simulink model "Auto_Coffee2"  (R2017a)
settings: Solver=FixedStepAuto  StartTime=0.0  StopTime=25  FixedStep=0.2  RelTol=1e-3
undefined symbols (not defined in the file): sigbuilder_block
libraries: nesl_utility x12, fl_lib x9
settings Model: Creator=Administrator  LastModifiedBy=Administrator
settings OptimizationCC: DefaultParameterBehavior=Inlined  UseDivisionForNetSlopeComputation=on  UseFloatMulNetSlope=on  InlineInvariantSignals=on  PassReuseOutputArgsAs=Individual arguments  ZeroExternalMemoryAtStartup=off  ZeroInternalMemoryAtStartup=off  NoFixptDivByZeroProtection=on  EfficientFloat2IntCast=on  LifeSpan=1
settings DebuggingCC: ParameterTunabilityLossMsg=error
settings HardwareCC: ProdBitPerPointer=32  ProdBitPerSizeT=32  ProdBitPerPtrDiffT=32  ProdLargestAtomicInteger=Long  ProdWordSize=32  ProdHWDeviceType=ARM Compatible->ARM 7
settings SFSimCC: MATLABDynamicMemAlloc=off
settings RTWCC: SystemTargetFile=ert.tlc  TemplateMakefile=ert_default_tmf  Description=Embedded Coder  GenerateReport=on  IncludeHyperlinkInReport=on  LaunchReport=on  GenerateTraceInfo=on  GenerateTraceReport=on  GenerateTraceReportSl=on  GenerateTraceReportSf=on  GenerateTraceReportEml=on  GenerateCodeMetricsReport=on
settings CodeAppCC: ForceParamTrailComments=on  IgnoreCustomStorageClasses=off  OperatorAnnotations=on  SimulinkDataObjDesc=on  SFDataObjDesc=on  MATLABFcnDesc=on  CustomSymbolStrGlobalVar=rt$N$M  CustomSymbolStrType=$N$M  CustomSymbolStrFcn=$N$M$F  CustomSymbolStrMacro=$N$M  InsertBlockDesc=on  MATLABSourceComments=on
settings ERTTargetCC: TargetLangStandard=C99 (ISO)  GenerateSampleERTMain=on  IncludeMdlTerminateFcn=off  CombineSignalStateStructs=on  SupportComplex=off  SupportContinuousTime=on  SupportNonInlinedSFcns=on  InlinedParameterPlacement=NonHierarchical  ERTCustomFileTemplate=example_file_process.tlc  ERTFilePackagingFormat=CompactWithDataFile

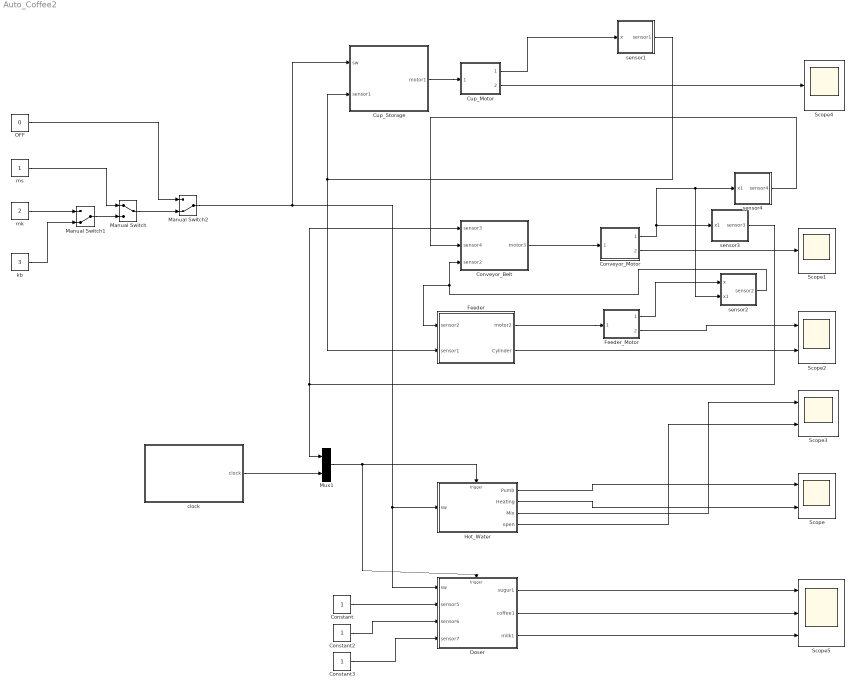
== system Auto_Coffee2 ==
  Constant : Constant
  Constant2 : Constant
  Constant3 : Constant
  Conveyor_Belt : Stateflow chart  TreatAsAtomicUnit=on
  Conveyor_Motor : Subsystem
  Cup_Motor : Subsystem
  Cup_Storage : Stateflow chart  TreatAsAtomicUnit=on
  Doser : Stateflow chart  TreatAsAtomicUnit=on
  Feeder : Stateflow chart  TreatAsAtomicUnit=on
  Feeder_Motor : Subsystem
  Hot_Water : Stateflow chart  TreatAsAtomicUnit=on
  Manual Switch : ManualSwitch
  Manual Switch1 : ManualSwitch  CurrentSetting=0
  Manual Switch2 : ManualSwitch  CurrentSetting=0
  Mux1 : Mux  Inputs=2
  OFF : Constant  Value=0
  Scope : Scope  NumInputPorts=2
  Scope1 : Scope
  Scope2 : Scope  NumInputPorts=2
  Scope3 : Scope  NumInputPorts=2
  Scope4 : Scope
  Scope5 : Scope  NumInputPorts=3
  clock : Subsystem  Tag=STV Subsys  LoadFcn=sigbuilder_block('load');  StartFcn=sigbuilder_block('start');  StopFcn=sigbuilder_block('stop');  ClipboardFcn=sigbuilder_block('clipboard');  mask(Sigbuilder block){tuvar=[0:10]}
      mask help: Simulink:masks:SigbuilderBlock_MD
      mask init:
      | if ~strcmp(get_param(bdroot(gcbh),'SimulationStatus'),'stopped') tuvar = sigbuilder_block('maskInit'); end
      settings: CopyFcn=sigbuilder_block('copy');  DeleteFcn=sigbuilder_block('delete');  ModelCloseFcn=sigbuilder_block('modelClose');  PreSaveFcn=sigbuilder_block('preSave');  PauseFcn=sigbuilder_block('pause');  ContinueFcn=sigbuilder_block('continue');  NameChangeFcn=sigbuilder_block('namechange');  OpenFcn=sigbuilder_block('open',[527.25 182.25 550.5 358.5 ]);  CloseFcn=sigbuilder_block('close');
      mask Display: plot(0, 0, 100, 100,[2, 2, 32, 32, 2], [68, 8, 8, 68, 68],[32, 2], [38, 38], [32, 19, 2],[53, 60, 44], [32, 17, 17, 2],[16, 16, 31, 31]);txt = getActiveGroup(gcbh);text(2, 100, txt,'verticalAlignment', 'top');
  kb : Constant  Value=3
  mk : Constant  Value=2
  ms : Constant
  sensor1 : Stateflow chart  TreatAsAtomicUnit=on
  sensor2 : Stateflow chart  TreatAsAtomicUnit=on
  sensor3 : Stateflow chart  TreatAsAtomicUnit=on
  sensor4 : Stateflow chart  TreatAsAtomicUnit=on
  wires:
  Hot_Water/1(Pumb) -> Scope/1
  Hot_Water/2(Heating) -> Scope/2
  Conveyor_Belt/1(motor3) -> Conveyor_Motor/1(motor3)
  Feeder/1(motor2) -> Feeder_Motor/1(motor2)
  Feeder/2(Cylinder) -> Scope2/2
  Cup_Storage/1(motor1) -> Cup_Motor/1(motor3)
  Constant/1 -> Doser/2(sensor5)
  Constant3/1 -> Doser/4(sensor7)
  Constant2/1 -> Doser/3(sensor6)
  clock/1(clock) -> Mux1/2
  Mux1/1 -> Hot_Water/Trigger, Doser/Trigger
  Manual Switch/1 -> Manual Switch2/2
  Manual Switch1/1 -> Manual Switch/2
  OFF/1 -> Manual Switch2/1
  ms/1 -> Manual Switch/1
  mk/1 -> Manual Switch1/1
  kb/1 -> Manual Switch1/2
  Doser/1(sugur1) -> Scope5/1
  Doser/2(coffee1) -> Scope5/2
  Doser/3(milk1) -> Scope5/3
  Conveyor_Motor/1(position) -> sensor2/2(x1), sensor4/1(x1), sensor3/1(x1)
  sensor4/1(sensor4) -> Conveyor_Belt/2(sensor4)
  Feeder_Motor/1(position) -> sensor2/1(x)
  sensor2/1(sensor2) -> Feeder/1(sensor2), Conveyor_Belt/3(sensor2)
  Cup_Motor/1(position) -> sensor1/1(x)
  sensor1/1(sensor1) -> Feeder/2(sensor1), Cup_Storage/2(sensor1)
  sensor3/1(sensor3) -> Mux1/1, Conveyor_Belt/1(sensor3)
  Manual Switch2/1 -> Hot_Water/1(sw), Doser/1(sw), Cup_Storage/1(sw)
  Hot_Water/3(Mix) -> Scope3/1
  Hot_Water/4(open) -> Scope3/2
  Feeder_Motor/2(scope1) -> Scope2/1
  Conveyor_Motor/2(scope1) -> Scope1/1
  Cup_Motor/2(scope1) -> Scope4/1

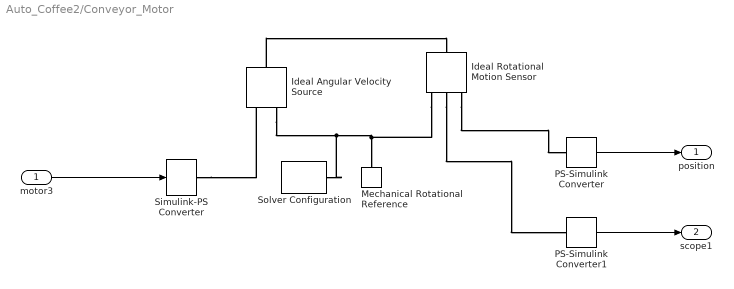
== system Auto_Coffee2/Conveyor_Motor ==
  motor3 : Inport
  Ideal Angular Velocity Source : fl_lib/Mechanical/Mechanical Sources/Ideal Angular Velocity Source
  Ideal Rotational Motion Sensor : fl_lib/Mechanical/Mechanical Sensors/Ideal Rotational Motion Sensor  offset=0 rad
  Mechanical Rotational Reference : fl_lib/Mechanical/Rotational Elements/Mechanical Rotational Reference
  PS-Simulink Converter : nesl_utility/PS-Simulink Converter  PhysicalDomain=network_engine_domain  SubClassName=ps_output  LeftPortType=input  RightPortType=output  PseudoPeriodic=off  Frequencies=[]  Unit=1  AffineConversion=off
  PS-Simulink Converter1 : nesl_utility/PS-Simulink Converter  PhysicalDomain=network_engine_domain  SubClassName=ps_output  LeftPortType=input  RightPortType=output  PseudoPeriodic=off  Frequencies=[]  Unit=1  AffineConversion=off
  Simulink-PS Converter : nesl_utility/Simulink-PS Converter  PhysicalDomain=network_engine_domain  SubClassName=ps_input  LeftPortType=input  RightPortType=output  PseudoPeriodic=off  Frequencies=[]  NoiseDistribution=none  NoiseParameters=[]  Unit=1  AffineConversion=off  FilteringAndDerivatives=zero  SimscapeFilterOrder=1  InputFilterTimeConstant=0.001  UdotUserProvided=1
  Solver Configuration : nesl_utility/Solver Configuration  PhysicalDomain=network_engine_domain  SubClassName=solver  LeftPortType=input  RightPortType=generic  Accelerate=off  Tones=[]  Harmonics=[]  SimulateNoise=off  Profile=off  UseLocalSampling=off  EnableSwitchedLinearOptims=on  FrequencyDomain=off  UseCCode=off  RelTol=0.001  AbsTol=1e-06  MinStep=1e-09  ToWorkspace=off  RevertToSquareIcSolve=off  NumHomotopyIterations=100  PhasorMode=off  PhasorModeNumHarmonics=1  OverrideAbsTol=off  DoDC=off  ResidualTolerance=1e-09  UseLocalSolver=off  LocalSolverChoice=NE_BACKWARD_EULER_ADVANCER  LocalSolverSampleTime=0.001  DoFixedCost=off  MaxNonlinIter=3  MaxModeIter=2  LinearAlgebra=Sparse  DelaysMemoryBudget=1024  AutomaticFiltering=on  FilteringTimeConstant=0.001
  position : Outport
  scope1 : Outport  Port=2
  wires:
  motor3/1 -> Simulink-PS Converter/1
  PS-Simulink Converter/1 -> position/1
  PS-Simulink Converter1/1 -> scope1/1
  connections:
  Ideal Angular Velocity Source/RConn2 -- Solver Configuration/RConn1 -- Ideal Rotational Motion Sensor/RConn1 -- Mechanical Rotational Reference/LConn1
  Ideal Angular Velocity Source/LConn1 -- Ideal Rotational Motion Sensor/LConn1
  Simulink-PS Converter/RConn1 -- Ideal Angular Velocity Source/RConn1
  Ideal Rotational Motion Sensor/RConn3 -- PS-Simulink Converter/LConn1
  Ideal Rotational Motion Sensor/RConn2 -- PS-Simulink Converter1/LConn1

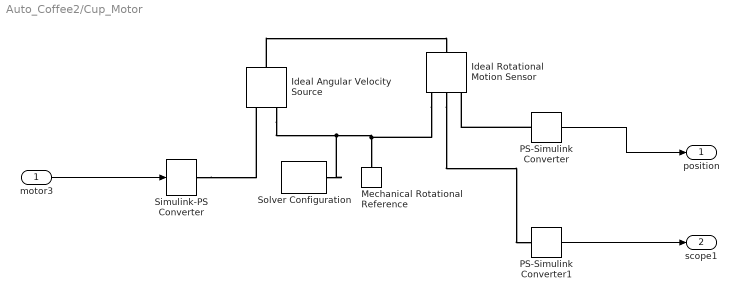
== system Auto_Coffee2/Cup_Motor ==
  motor3 : Inport
  Ideal Angular Velocity Source : fl_lib/Mechanical/Mechanical Sources/Ideal Angular Velocity Source
  Ideal Rotational Motion Sensor : fl_lib/Mechanical/Mechanical Sensors/Ideal Rotational Motion Sensor  offset=0 rad
  Mechanical Rotational Reference : fl_lib/Mechanical/Rotational Elements/Mechanical Rotational Reference
  PS-Simulink Converter : nesl_utility/PS-Simulink Converter  PhysicalDomain=network_engine_domain  SubClassName=ps_output  LeftPortType=input  RightPortType=output  PseudoPeriodic=off  Frequencies=[]  Unit=1  AffineConversion=off
  PS-Simulink Converter1 : nesl_utility/PS-Simulink Converter  PhysicalDomain=network_engine_domain  SubClassName=ps_output  LeftPortType=input  RightPortType=output  PseudoPeriodic=off  Frequencies=[]  Unit=1  AffineConversion=off
  Simulink-PS Converter : nesl_utility/Simulink-PS Converter  PhysicalDomain=network_engine_domain  SubClassName=ps_input  LeftPortType=input  RightPortType=output  PseudoPeriodic=off  Frequencies=[]  NoiseDistribution=none  NoiseParameters=[]  Unit=1  AffineConversion=off  FilteringAndDerivatives=zero  SimscapeFilterOrder=1  InputFilterTimeConstant=0.001  UdotUserProvided=1
  Solver Configuration : nesl_utility/Solver Configuration  PhysicalDomain=network_engine_domain  SubClassName=solver  LeftPortType=input  RightPortType=generic  Accelerate=off  Tones=[]  Harmonics=[]  SimulateNoise=off  Profile=off  UseLocalSampling=off  EnableSwitchedLinearOptims=on  FrequencyDomain=off  UseCCode=off  RelTol=0.001  AbsTol=1e-06  MinStep=1e-09  ToWorkspace=off  RevertToSquareIcSolve=off  NumHomotopyIterations=100  PhasorMode=off  PhasorModeNumHarmonics=1  OverrideAbsTol=off  DoDC=off  ResidualTolerance=1e-09  UseLocalSolver=off  LocalSolverChoice=NE_BACKWARD_EULER_ADVANCER  LocalSolverSampleTime=0.001  DoFixedCost=off  MaxNonlinIter=3  MaxModeIter=2  LinearAlgebra=Sparse  DelaysMemoryBudget=1024  AutomaticFiltering=on  FilteringTimeConstant=0.001
  position : Outport
  scope1 : Outport  Port=2
  wires:
  PS-Simulink Converter/1 -> position/1
  motor3/1 -> Simulink-PS Converter/1
  PS-Simulink Converter1/1 -> scope1/1
  connections:
  Ideal Angular Velocity Source/RConn2 -- Solver Configuration/RConn1 -- Ideal Rotational Motion Sensor/RConn1 -- Mechanical Rotational Reference/LConn1
  Ideal Angular Velocity Source/LConn1 -- Ideal Rotational Motion Sensor/LConn1
  PS-Simulink Converter/LConn1 -- Ideal Rotational Motion Sensor/RConn3
  Simulink-PS Converter/RConn1 -- Ideal Angular Velocity Source/RConn1
  Ideal Rotational Motion Sensor/RConn2 -- PS-Simulink Converter1/LConn1

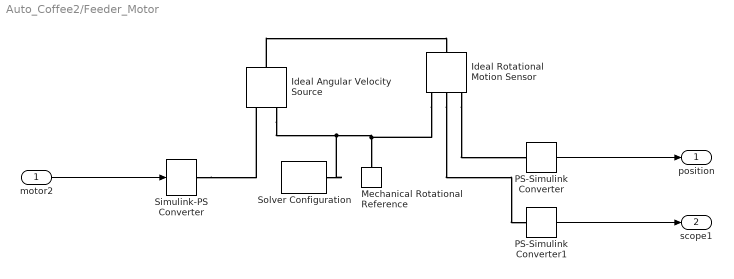
== system Auto_Coffee2/Feeder_Motor ==
  motor2 : Inport
  Ideal Angular Velocity Source : fl_lib/Mechanical/Mechanical Sources/Ideal Angular Velocity Source
  Ideal Rotational Motion Sensor : fl_lib/Mechanical/Mechanical Sensors/Ideal Rotational Motion Sensor  offset=0 rad
  Mechanical Rotational Reference : fl_lib/Mechanical/Rotational Elements/Mechanical Rotational Reference
  PS-Simulink Converter : nesl_utility/PS-Simulink Converter  PhysicalDomain=network_engine_domain  SubClassName=ps_output  LeftPortType=input  RightPortType=output  PseudoPeriodic=off  Frequencies=[]  Unit=1  AffineConversion=off
  PS-Simulink Converter1 : nesl_utility/PS-Simulink Converter  PhysicalDomain=network_engine_domain  SubClassName=ps_output  LeftPortType=input  RightPortType=output  PseudoPeriodic=off  Frequencies=[]  Unit=1  AffineConversion=off
  Simulink-PS Converter : nesl_utility/Simulink-PS Converter  PhysicalDomain=network_engine_domain  SubClassName=ps_input  LeftPortType=input  RightPortType=output  PseudoPeriodic=off  Frequencies=[]  NoiseDistribution=none  NoiseParameters=[]  Unit=1  AffineConversion=off  FilteringAndDerivatives=zero  SimscapeFilterOrder=1  InputFilterTimeConstant=0.001  UdotUserProvided=1
  Solver Configuration : nesl_utility/Solver Configuration  PhysicalDomain=network_engine_domain  SubClassName=solver  LeftPortType=input  RightPortType=generic  Accelerate=off  Tones=[]  Harmonics=[]  SimulateNoise=off  Profile=off  UseLocalSampling=off  EnableSwitchedLinearOptims=on  FrequencyDomain=off  UseCCode=off  RelTol=0.001  AbsTol=1e-06  MinStep=1e-09  ToWorkspace=off  RevertToSquareIcSolve=off  NumHomotopyIterations=100  PhasorMode=off  PhasorModeNumHarmonics=1  OverrideAbsTol=off  DoDC=off  ResidualTolerance=1e-09  UseLocalSolver=off  LocalSolverChoice=NE_BACKWARD_EULER_ADVANCER  LocalSolverSampleTime=0.001  DoFixedCost=off  MaxNonlinIter=3  MaxModeIter=2  LinearAlgebra=Sparse  DelaysMemoryBudget=1024  AutomaticFiltering=on  FilteringTimeConstant=0.001
  position : Outport
  scope1 : Outport  Port=2
  wires:
  motor2/1 -> Simulink-PS Converter/1
  PS-Simulink Converter/1 -> position/1
  PS-Simulink Converter1/1 -> scope1/1
  connections:
  Ideal Angular Velocity Source/RConn2 -- Solver Configuration/RConn1 -- Ideal Rotational Motion Sensor/RConn1 -- Mechanical Rotational Reference/LConn1
  Ideal Angular Velocity Source/LConn1 -- Ideal Rotational Motion Sensor/LConn1
  Simulink-PS Converter/RConn1 -- Ideal Angular Velocity Source/RConn1
  Ideal Rotational Motion Sensor/RConn3 -- PS-Simulink Converter/LConn1
  Ideal Rotational Motion Sensor/RConn2 -- PS-Simulink Converter1/LConn1

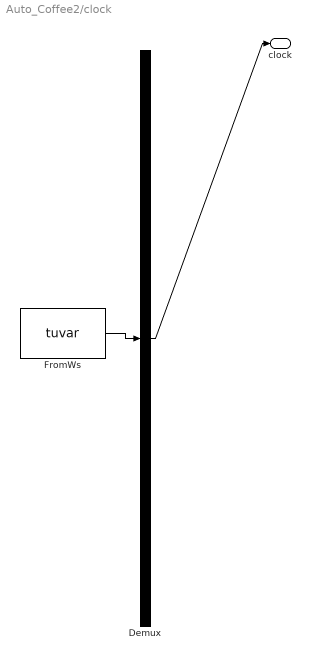
== system Auto_Coffee2/clock ==
  Demux : Demux  Tag=STV Demux  Outputs=1
  FromWs : FromWorkspace  Tag=STV FromWs  VariableName=tuvar  SampleTime=0
      SigBuilderData=|
      | common.afterFinalStr = 'Extrapolate'
      | common.sampleTime = 0
      | dataSet.timeRange = [0 25]
      | dataSet.name = 'Group 1'
      | sbobj.Groups.Name = 'Group 1'
      | sbobj.Groups.Signals.Name = 'clock'
      | sbobj.Groups.Signals.XData = [0 0.2 0.2 0.4 0.4 0.6 0.6 0.8 0.8 1 1 1.2 1.2 1.4 1.4 1.6 1.6 1.8 1.8 2 2 2.2 2.2 2.4 2.4 2.6 2.6 2.8 2.8 3 3 3.2 3.2 3.4 3.4 3.6 3.6 3.8 3.8 4 4 4.2 4.2 4.4 4.4 4.6 4.6 4.8 4.8 5 5 5.2 5.2 5.4 5.4 5.6 5.6 5.8 5.8 6 6 6.2 6.2 6.4 6.4 6.6 6.6 6.8 6.8 7 7 7.2 7.2 7.4 7.4 7.6 7.6 7.8 7.8 8 8 8.2 8.2 8.4 8.4 8.6 8.6 8.8 8.8 9 9 9.2 9.2 9.4 9.4 9.6 9.6 9.8 9.8 10 10 10.2 10.2 10.4 10.4 10.6 10.6 10.8 10.8 11 11 11.2 11.2 11.4 11.4 11.6 11.6 11.8 11.8 12 12 12.2 12.2 12.4 12.4 12.6 12.6 12.8 12.8 13 13 13.2 13.2 13.4 13.4 13.6 13.6 13.8 13.8 14 14 14.2 14.2 14.4 14.4 14.6 14.6 14.8 14.8 15 15 15.2 15.2 15.4 15.4 15.6 15.6 15.8 15.8 16 16 16.2 16.2 16.4 16.4 16.6 16.6 16.8 16.8 17 17 17.2 17.2 17.4 17.4 17.6 17.6 17.8 17.8 18 18 18.2 18.2 18.4 18.4 18.6 18.6 18.8 18.8 19 19 19.2 19.2 19.4 19.4 19.6 19.6 19.8 19.8 20 20 20.2 20.2 20.4 20.4 20.6 20.6 20.8 20.8 21 21 21.2 21.2 21.4 21.4 21.6 21.6 21.8 21.8 22 22 22.2 22.2 22.4 22.4 22.6 22.6 22.8 22.8 23 23 23.2 23.2 23.4 23.4 23.6 23.6 23.8 23.8 24 24 24.2 24.2 24.4 24.4 24.6 24.6 24.8 24.8 25]
      | sbobj.Groups.Signals.YData = [2 2 0 0 2 2 0 0 2 2 0 0 2 2 0 0 2 2 0 0 2 2 0 0 2 2 0 0 2 2 0 0 2 2 0 0 2 2 0 0 2 2 0 0 2 2 0 0 2 2 0 0 2 2 0 0 2 2 0 0 2 2 0 0 2 2 0 0 2 2 0 0 2 2 0 0 2 2 0 0 2 2 0 0 2 2 0 0 2 2 0 0 2 2 0 0 2 2 0 0 2 2 0 0 2 2 0 0 2 2 0 0 2 2 0 0 2 2 0 0 2 2 0 0 2 2 0 0 2 2 0 0 2 2 0 0 2 2 0 0 2 2 0 0 2 2 0 0 2 2 0 0 2 2 0 0 2 2 0 0 2 2 0 0 2 2 0 0 2 2 0 0 2 2 0 0 2 2 0 0 2 2 0 0 2 2 0 0 2 2 0 0 2 2 0 0 2 2 0 0 2 2 0 0 2 2 0 0 2 2 0 0 2 2 0 0 2 2 0 0 2 2 0 0 2 2 0 0 2 2 0 0 2 2 0 0 2 2 0 0 2 2 0 0 2 2 0 0 2 2]
      | sbobj.Groups.TimeRange = [0 25]
  clock : Outport  Tag=STV Outport
  wires:
  FromWs/1 -> Demux/1
  Demux/1 -> clock/1

== stateflow chart Auto_Coffee2/Conveyor_Belt ==
  state ON
    state motor_on
      en:motor3=1;
    state motor_off
      en:motor3=0;
    (default) -> motor_on
    motor_on -> motor_off : [sensor3==1]
    motor_off -> motor_on : after(10,sec)
  state OFF
    en:motor3=0;
  OFF -> ON : [sensor4==0&&sensor2==1]
  ON -> OFF : [sensor4==1&&sensor2==0]
  (default) -> OFF
  data: sensor3 input; sensor4 input; sensor2 input; motor3 output

== stateflow chart Auto_Coffee2/Feeder ==
  state On
    en:motor2=1
  state OFF
    en:motor2=0
  state On1
    en:Cylinder=1
  state Off2
    en:Cylinder=0
  state OFF2
    en:motor2=0
  (default) -> OFF
  OFF -> On : [sensor1==1]
  On1 -> Off2 : after(1,sec)
  OFF2 -> On1 : after(1,sec)
  On -> OFF2 : [sensor2==1]
  data: motor2 output; sensor2 input; sensor1 input; Cylinder output

== stateflow chart Auto_Coffee2/Hot_Water ==
  settings: executeAtInitialization=1
  state PowerOn
    state Pumb [parallel]
      settings: executionOrder=1
      state On
        en:Pumb=1;
        pumb=1;
      state Off
        en:Pumb=0;
        pumb=0;
      PowerOn.Pumb.On -> PowerOn.Pumb.Off : after(10,sec)
      PowerOn.Pumb.Off -> PowerOn.Pumb.On : sensor3
      (default) -> PowerOn.Pumb.Off
    state Heating [parallel]
      settings: executionOrder=2
      state On
        en:Heating=1;
      state Off
        en:Heating=0;
      PowerOn.Heating.On -> PowerOn.Heating.Off : after(10,sec)
      PowerOn.Heating.Off -> PowerOn.Heating.On : sensor3
      (default) -> PowerOn.Heating.Off
    state mix [parallel]
      settings: executionOrder=3
      state off
        en:Mix=0;
        open=0;
      state wait
        en:Mix=0;
        open=0;
      state on
        en:Mix=0;
        open=1;
      state mix
        en:Mix=1;
      (default) -> off
      off -> wait : [pumb==1]
      on -> off : after(3,sec)
      wait -> PowerOn.mix.mix : after(5,sec)
      PowerOn.mix.mix -> on : after(2,sec)
  state PowerOff
  PowerOff -> PowerOn : [sw~=0]
  PowerOn -> PowerOff : [sw==0]
  (default) -> PowerOff
  data: sw input; Pumb output; Heating output; Mix output; open output; pumb local
  events: sensor3 input RISING_EDGE_EVENT; clock input RISING_EDGE_EVENT

== stateflow chart Auto_Coffee2/Cup_Storage ==
  state on
    state motor_off
      en:motor1=0;
    state motor_on
      en:motor1=1;
      flag=1;
    motor_off -> motor_on : [sensor1==0&&flag==0]
    motor_on -> motor_off : after(1,sec)
    (default) -> motor_off
  state off
    en:motor1=0;
    flag=0;
  off -> on : [sw~=0]
  on -> off : [sw==0]
  (default) -> off
  data: sw input; motor1 output; sensor1 input; flag local

== stateflow chart Auto_Coffee2/Doser ==
  settings: executeAtInitialization=1
  state on
    state coffee [parallel]
      settings: executionOrder=1
      state on
        en:coffee1=1
      state off
        en:coffee1=0
      on.coffee.on -> on.coffee.off : [sensor7==0||after(10,sec)]
      on.coffee.off -> on.coffee.on : [sw~=0&&sensor3&&sensor7==1]
      (default) -> on.coffee.off
    state milk [parallel]
      settings: executionOrder=2
      state on
        en:milk1=1
      state off
        en:milk1=0
      on.milk.on -> on.milk.off : [sensor5==0||after(10,sec)]
      on.milk.off -> on.milk.on : [(sw==2||sw==3)&&sensor3&&sensor5]
      (default) -> on.milk.off
    state sugur [parallel]
      settings: executionOrder=3
      state on
        en:sugur1=1
      state off
        en:sugur1=0
      on.sugur.on -> on.sugur.off : [sensor6==0||after(10,sec)]
      on.sugur.off -> on.sugur.on : [sw==3&&sensor3&&sensor6]
      (default) -> on.sugur.off
  state off
    en:coffee1=0;
    milk1=0;
    sugur1=0;
  on -> off : [sw==0]
  off -> on : [sw~=0]
  (default) -> off
  data: sw input; sensor5 input; sensor6 input; sensor7 input; sugur1 output; coffee1 output; milk1 output
  events: sensor3 input RISING_EDGE_EVENT; clock input RISING_EDGE_EVENT

== stateflow chart Auto_Coffee2/sensor4 ==
  state state
    state state1
      en:sensor4=0;
    state state2
      en:sensor4=1;
    state1 -> state2 : [abs(x1-9)<1e-6]
    state2 -> state1 : [x1~=9]
    (default) -> state1
  (default) -> state
  data: sensor4 output; x1 input

== stateflow chart Auto_Coffee2/sensor2 ==
  state state
    state state1
      en:sensor2=0;
    state state2
      en:sensor2=1;
    state state
      en:sensor2=0
    state1 -> state2 : [abs(x-2)<1e-6]
    state2 -> state.state : [abs(x1-0)>1e-1]
    (default) -> state1
  (default) -> state
  data: x input; sensor2 output; x1 input

== stateflow chart Auto_Coffee2/sensor1 ==
  state state
    state state1
      en:sensor1=0;
    state state2
      en:sensor1=1;
    state state
      en:sensor1=0
    state1 -> state2 : [abs(x-1)<1e-6]
    state2 -> state.state : after(1,sec)
    (default) -> state1
  (default) -> state
  data: x input; sensor1 output

== stateflow chart Auto_Coffee2/sensor3 ==
  state state
    state state1
      en:sensor3=0;
    state state2
      en:sensor3=1;
    state1 -> state2 : [abs(x1-6.6)<1e-6]
    state2 -> state1 : after(10,sec)
    (default) -> state1
  (default) -> state
  data: sensor3 output; x1 input
